simulink model "generic_IVS"  (R2024a)
settings: Solver=FixedStepDiscrete  StartTime=0.0  StopTime=inf  FixedStep=0.001  RelTol=1e-3  EnableMultiTasking=on
model workspace (MAT data in the model file):
  APPROACH = [-49.2532697283 -46.8560638421 -44.4231792578 -41.9812023919 -38.6885385845 -35.362557161 -32.0241539117 -28.6853351363 -25.3485360015 -22.0129625698 -18.6780310991 -15.3435011563 ... (76 elements, 38x2)]
  LANE_LEN = [284; 276; 267]
  LANE_XY = [59.0003214677 62.3317238784 65.6577746803 68.9711287644 72.2614514234 75.5172879138 77.9296982442 80.3117765819 82.6592727002 84.9682672017 87.2351542049 89.4565910317 ... (1704 elements, 284x2x3)]
  N_LANE = 3
  PARK_OCC = [1 1 1 1 1 1 1 1 1 1 1 1 ... (40000 elements, 200x200)]
  WB = 2.9
  branch_lane = 3
  branch_x = -49.2532697283
  branch_y = 17.3349288561
  cruise_lane = 1
  entrance_x = 6
  entrance_y = -36.6
  lane_width = 3.5
  park_goal = [21.4; -44.3; 1.57079632679]
  toll_lane = 1
  toll_post = 20
  toll_pre = 45
  toll_station = 202.6
  toll_x = -176.17
  toll_y = -85.66
  v_cruise = 11
  v_park = 2.78
  waypoints = [-81.8048181182 -79.1416974235 -76.4199514846 -73.3097017696 -70.5703457405 -67.625901331 -64.4903894371 -61.1945301864 -57.8351626085 -54.4642235015 -51.0966947204 -47.7361432477 ... (1754 elements, 877x2)]
libraries: CarMaker4SL x57, simulink x1
(part 2 of 4)

== system generic_IVS/CarMaker ==
  note: Do Not Modify !!
  note: Modify !!
  CM_FIRST : Subsystem
  CM_LAST : Subsystem
  DrivMan : Subsystem
  Ground : Ground
  IPG Vehicle : Subsystem
  IVS_Control : Subsystem
  Subsystem : Subsystem
  Terminator : Terminator
  VehicleControl : Subsystem
  wires:
  DrivMan/2(DrivMan.Out) -> VehicleControl/2(DrivMan.In)
  DrivMan/1(Sync_Out) -> VehicleControl/1(Sync_In)
  CM_FIRST/2(Env.Misc) -> DrivMan/2(Env.Misc)
  CM_FIRST/1(Sync_Out) -> DrivMan/1(Sync_In)
  CM_LAST/1(Sync_Out) -> Terminator/1
  Ground/1 -> CM_FIRST/1(Sync_In)
  IPG Vehicle/1(Sync_Out) -> CM_LAST/1(Sync_In)
  VehicleControl/1(Sync_Out) -> IPG Vehicle/1(Sync_In)
  VehicleControl/3(VhclCtrl.Steering) -> IPG Vehicle/3(VhclCtrl.Steering)
  VehicleControl/4(Vhcl.Wheel.In) -> IPG Vehicle/4(Vhcl.Wheel.In)
  VehicleControl/5(Vhcl.Misc) -> IPG Vehicle/5(Vhcl.Misc)
  VehicleControl/6(VhclCtrl.Brake) -> IPG Vehicle/6(VhclCtrl.Brake)
  VehicleControl/7(VhclCtrl.PT) -> IPG Vehicle/7(VhclCtrl.PT)
  VehicleControl/2(Vhcl.Model.Source) -> IPG Vehicle/2(Vhcl.Model.Source)

== system generic_IVS/Open CarMaker GUI ==
  S-Function : S-Function  FunctionName=cm_gui  SFunctionDeploymentMode=off  EnableBusSupport=off

== system generic_IVS/CarMaker/CM_FIRST ==
  Sync_In : Inport
  BusCreator1 : BusCreator  Inputs=8
  BusCreator2 : BusCreator  Inputs=6
  Demux1 : Demux  Outputs=14
      settings: DisplayOption=none
  Environment : S-Function  FunctionName=CM_Sfun  Parameters='Environment'  SFunctionDeploymentMode=off  EnableBusSupport=off
  IoIn : S-Function  FunctionName=CM_Sfun  Parameters='IoIn'  SFunctionDeploymentMode=off  EnableBusSupport=off
  Terminator : Terminator
  Sync_Out : Outport  VectorParamsAs1DForOutWhenUnconnected=off
  Env.Misc : Outport  Port=2  VectorParamsAs1DForOutWhenUnconnected=off
  wires:
  BusCreator2/1 -> Terminator/1  "IF Environment (in)"
  BusCreator1/1 -> Env.Misc/1
  Demux1/14 -> BusCreator2/6  "Env sRoad"
  Demux1/13 -> BusCreator2/5  "Env PoI_GCS Elev"
  Demux1/12 -> BusCreator2/4  "Env PoI_GCS Lat"
  Demux1/11 -> BusCreator2/3  "Env PoI_GCS Long"
  Demux1/10 -> BusCreator2/2  "Env Time"
  Demux1/9 -> BusCreator2/1  "Env yDay"
  Demux1/8 -> BusCreator1/8  "Env WindVel_tot z"
  Demux1/7 -> BusCreator1/7  "Env WindVel_tot y"
  Demux1/6 -> BusCreator1/6  "Env WindVel_tot x"
  Demux1/5 -> BusCreator1/5  "Env SolarRadiation"
  Demux1/4 -> BusCreator1/4  "Env AirHumidity"
  Demux1/3 -> BusCreator1/3  "Env AirPressure"
  Demux1/2 -> BusCreator1/2  "Env AirDensity"
  Demux1/1 -> BusCreator1/1  "Env Temperature"
  Environment/2 -> Demux1/1
  Environment/1 -> Sync_Out/1
  IoIn/1 -> Environment/1
  Sync_In/1 -> IoIn/1

== system generic_IVS/CarMaker/CM_LAST ==
  Sync_In : Inport
  CM_User : S-Function  FunctionName=CM_Sfun  Parameters='CM_User'  SFunctionDeploymentMode=off  EnableBusSupport=off
  IoOut : S-Function  FunctionName=CM_Sfun  Parameters='IoOut'  SFunctionDeploymentMode=off  EnableBusSupport=off
  Sync_Out : Outport  VectorParamsAs1DForOutWhenUnconnected=off
  wires:
  IoOut/1 -> Sync_Out/1
  CM_User/1 -> IoOut/1
  Sync_In/1 -> CM_User/1

== system generic_IVS/CarMaker/DrivMan ==
  note: There's rarely a reason to override DrivMan signals.
      | Use the VehicleControl interface for this purpose.
  Sync_In : Inport
  Env.Misc : Inport  Port=2
  BusCreator : BusCreator  Inputs=20
  Demux : Demux  Outputs=20
      settings: DisplayOption=none
  DrivMan : S-Function  FunctionName=CM_Sfun  Parameters='DrivMan'  SFunctionDeploymentMode=off  EnableBusSupport=off
  Sync_Out : Outport  VectorParamsAs1DForOutWhenUnconnected=off
  DrivMan.Out : Outport  Port=2  VectorParamsAs1DForOutWhenUnconnected=off
  wires:
  Demux/8 -> BusCreator/8  "DrivMan SelectorCtrl"
  Demux/7 -> BusCreator/7  "DrivMan UserSignal4"
  Demux/6 -> BusCreator/6  "DrivMan UserSignal3"
  Demux/5 -> BusCreator/5  "DrivMan UserSignal2"
  Demux/4 -> BusCreator/4  "DrivMan UserSignal1"
  Demux/3 -> BusCreator/3  "DrivMan UserSignal0"
  Demux/2 -> BusCreator/2  "DrivMan Key"
  Demux/1 -> BusCreator/1  "DrivMan SST"
  Env.Misc/1 -> DrivMan/2
  Sync_In/1 -> DrivMan/1
  DrivMan/1 -> Sync_Out/1
  BusCreator/1 -> DrivMan.Out/1
  DrivMan/2 -> Demux/1
  Demux/9 -> BusCreator/9  "DrivMan DigitalSelectorCtrl0"
  Demux/10 -> BusCreator/10  "DrivMan DigitalSelectorCtrl1"
  Demux/11 -> BusCreator/11  "DrivMan DigitalSelectorCtrl2"
  Demux/20 -> BusCreator/20  "DrivMan Steering Trq"
  Demux/19 -> BusCreator/19  "DrivMan Steering AngAcc"
  Demux/18 -> BusCreator/18  "DrivMan Steering AngVel"
  Demux/17 -> BusCreator/17  "DrivMan Steering Ang"
  Demux/16 -> BusCreator/16  "DrivMan Gas"
  Demux/15 -> BusCreator/15  "DrivMan Clutch"
  Demux/14 -> BusCreator/14  "DrivMan BrakePark"
  Demux/13 -> BusCreator/13  "DrivMan Brake"
  Demux/12 -> BusCreator/12  "DrivMan GearNo"

== system generic_IVS/CarMaker/IPG Vehicle ==
  Sync_In : Inport
  Vhcl.Model.Source : Inport  Port=2
  VhclCtrl.Steering : Inport  Port=3
  Vhcl.Wheel.In : Inport  Port=4
  Vhcl.Misc : Inport  Port=5
  VhclCtrl.Brake : Inport  Port=6
  VhclCtrl.PT : Inport  Port=7
  Brake : Subsystem
  CarAndTrailer : Subsystem
  PowerTrain : Subsystem
  Stop Simulation : Stop
  VehicleSource_BuiltIn : simulink/Logic and Bit Operations/Compare To Constant  relop=~=  const=1  OutDataTypeStr=boolean  ZeroCross=off
  Sync_Out : Outport  VectorParamsAs1DForOutWhenUnconnected=off
  wires:
  VhclCtrl.PT/1 -> PowerTrain/3(VhclCtrl.PT)
  Brake/1(Sync_Out) -> PowerTrain/1(Sync_In)
  CarAndTrailer/1(Sync_Out) -> Brake/1(Sync_In)
  CarAndTrailer/2(Brake.IF.In) -> Brake/2(Brake.IF.In)
  VhclCtrl.Brake/1 -> Brake/3(VhclCtrl.Brake)
  PowerTrain/1(Sync_Out) -> Sync_Out/1
  Vhcl.Misc/1 -> CarAndTrailer/4(Vhcl.Misc)
  Vhcl.Wheel.In/1 -> CarAndTrailer/3(Vhcl.Wheel.In)
  VhclCtrl.Steering/1 -> CarAndTrailer/2(VhclCtrl.Steering)
  Sync_In/1 -> CarAndTrailer/1(Sync_In)
  Vhcl.Model.Source/1 -> VehicleSource_BuiltIn/1
  VehicleSource_BuiltIn/1 -> Stop Simulation/1
  Brake/2(Vhcl.Wheel.PT) -> PowerTrain/2(Vhcl.Wheel.PT)

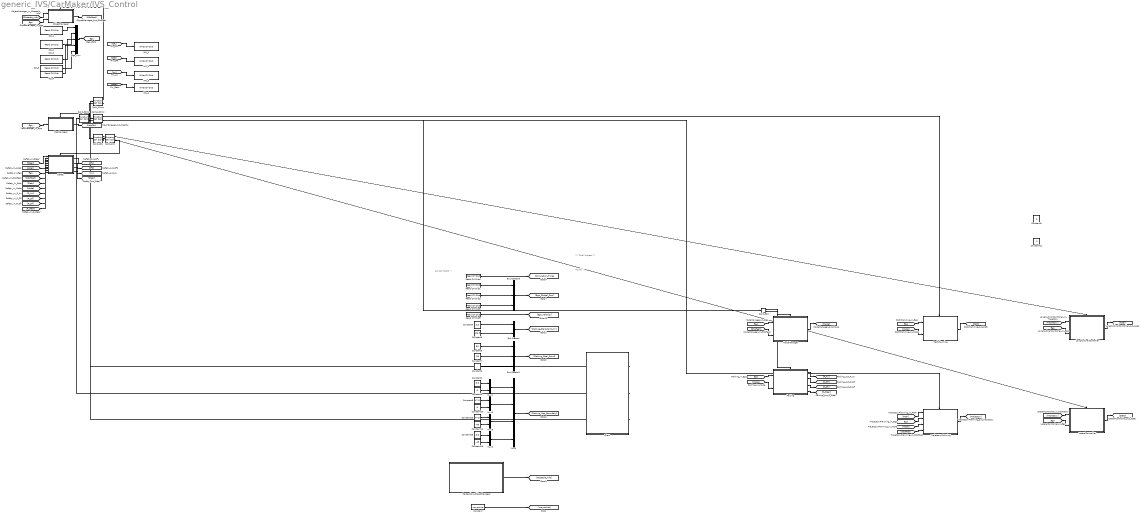
== system generic_IVS/CarMaker/IVS_Control ==
  note: Do Not Modify !!
  note: *** Final Project ***
  note: Modify !!
  Bus Creator : BusCreator  Inputs=2
  Bus Creator1 : BusCreator  Inputs=3
  Bus Creator3 : BusCreator  Inputs=3
  Chart : Stateflow chart  TreatAsAtomicUnit=on
  Constant : Constant  Value=waypoints
  Constant1 : Constant  Value=5.5
  Constant10 : Constant  Value=-4
  Constant11 : Constant  Value=-1
  Constant13 : Constant  Value=47.5
  Constant14 : Constant  Value=-45
  Constant15 : Constant  Value=5.5
  Constant16 : Constant  Value=-45
  Constant2 : Constant  Value=2*pi/3
  Constant3 : Constant
  Constant4 : Constant  Value=5.5
  Constant5 : Constant  Value=-36.5
  Constant6 : Constant  Value=35
  Constant7 : Constant  Value=-30
  Constant8 : Constant  Value=47.5
  Constant9 : Constant  Value=-4
  Ego_Mux : Mux  Inputs=5
  LateralController : Subsystem
  LongitudinalController : Subsystem
  MapManager : Subsystem
  ModeManager : Subsystem
  Mux{2,5,8..9} (4 alike) : Mux  Inputs=2
  Mux4 : Mux
  ObjectManager : Subsystem
  Parking : Subsystem
  PathPlanning : Subsystem
  Perception_ObjectManager : Subsystem
  RD_1 : CarMaker4SL/Read CM Dict  xname=Car.Fr1.tx  xsync=off  xstime=Continuous
  RD_2 : CarMaker4SL/Read CM Dict  xname=Car.Fr1.ty  xsync=off  xstime=Continuous
  RD_3 : CarMaker4SL/Read CM Dict  xname=Car.Fr1.rz  xsync=off  xstime=Continuous
  RD_4 : CarMaker4SL/Read CM Dict  xname=Car.v  xsync=off  xstime=Continuous
  RD_5 : CarMaker4SL/Read CM Dict  xname=Car.Road.sRoad  xsync=off  xstime=Continuous
  Read CM Dict1 : CarMaker4SL/Read CM Dict  xname=Car.Fr1.tx  xsync=off  xstime=Inherited
  Read CM Dict2 : CarMaker4SL/Read CM Dict  xname=Car.Fr1.ty  xsync=off  xstime=Inherited
  Read CM Dict3 : CarMaker4SL/Read CM Dict  xname=Car.Fr1.rz  xsync=off  xstime=Inherited
  Read CM Dict4 : CarMaker4SL/Read CM Dict  xname=Time  xsync=off  xstime=Inherited
  Read CM Dict5 : CarMaker4SL/Read CM Dict  xname=Car.v  xsync=off  xstime=Inherited
  Safety : Subsystem
  Split_100ms : FunctionCallSplit  IconShape=distinctive  NumOutputPorts=2  OutputPortLayout=default
  Split_10b : FunctionCallSplit  IconShape=distinctive  NumOutputPorts=2  OutputPortLayout=default
  Split_10c : FunctionCallSplit  IconShape=distinctive  NumOutputPorts=2  OutputPortLayout=default
  Split_10ms : FunctionCallSplit  IconShape=distinctive  NumOutputPorts=2  OutputPortLayout=default
  Split_50d : FunctionCallSplit  IconShape=distinctive  NumOutputPorts=2  OutputPortLayout=default
  Split_50ms : FunctionCallSplit  IconShape=distinctive  NumOutputPorts=2  OutputPortLayout=default
  TrajectoryPlanning : Subsystem
  WR_1 : CarMaker4SL/Write CM Dict  xname=Car.CFL.rz_ext  xsync=off
  WR_2 : CarMaker4SL/Write CM Dict  xname=Car.CFR.rz_ext  xsync=off
  WR_3 : CarMaker4SL/Write CM Dict  xname=AccelCtrl.DesiredAx  xsync=off
  WR_4 : CarMaker4SL/Write CM Dict  xname=DM.SelectorCtrl  xsync=off
  tag scope: Ego=global
  wires:
  Constant13/1 -> Mux8/1
  Perception_ObjectManager/1(Traffic_Info) -> [Obstacle_Info]
  Read CM Dict1/1 -> Bus Creator3/1  "Car_Fr1_tx"
  Read CM Dict3/1 -> Bus Creator3/3  "Car_Fr1_rz"
  Constant4/1 -> Bus Creator/1  "Parking_Start_Point_X"
  Read CM Dict4/1 -> [Simulation_Time]  "Time"
  Constant9/1 -> Mux2/2
  Bus Creator1/1 -> [Parking_Goal_Point]
  Mux8/1 -> Mux4/3
  Constant6/1 -> Bus Creator1/1  "Parking_Goal_Point_X"
  Constant1/1 -> Mux2/1
  Constant16/1 -> Mux9/2
  Read CM Dict2/1 -> Bus Creator3/2  "Car_Fr1_ty"
  Constant5/1 -> Bus Creator/2  "Parking_Start_Point_Y"
  Constant7/1 -> Bus Creator1/2  "Parking_Goal_Point_Y"
  Read CM Dict5/1 -> [Ego_Velocity]  "Car.v"
  Constant15/1 -> Mux9/1
  Constant10/1 -> Mux5/2
  Bus Creator3/1 -> [Ego_Global_Pos]
  Constant14/1 -> Mux8/2
  Bus Creator/1 -> [Parking_Start_Point_XY]
  Mux9/1 -> Mux4/4
  Mux2/1 -> Mux4/1
  Mux4/1 -> [Parking_Map_Boundary]
  Constant8/1 -> Mux5/1
  Constant2/1 -> Bus Creator1/3  "Parking_Goal_Point_Yaw"
  Mux5/1 -> Mux4/2
  Constant/1 -> [waypoints]
  Chart/1(do_Logic_10ms()) -> Split_10ms/1
  Chart/3(do_Logic_100ms()) -> Split_100ms/1
  RD_1/1 -> Ego_Mux/1
  RD_2/1 -> Ego_Mux/2
  RD_3/1 -> Ego_Mux/3
  RD_4/1 -> Ego_Mux/4
  Ego_Mux/1 -> [Ego]
  Chart/2(do_Logic_50ms()) -> Split_50ms/1
  [Ego] -> MapManager/1(Ego)
  MapManager/1(MapCtx) -> [MapCtx]
  [Trajectory] -> LateralController/1(Trajectory)
  [Ego] -> LateralController/2(Ego)
  LateralController/1(Steer) -> [Steer]
  [Trajectory] -> LongitudinalController/1(Trajectory)
  [Ego] -> LongitudinalController/2(Ego)
  LongitudinalController/1(Accel) -> [Accel]
  Split_50ms/1 -> MapManager/Trigger
  Split_100ms/1 -> PathPlanning/Trigger
  Split_100ms/2 -> TrajectoryPlanning/Trigger
  RD_5/1 -> Ego_Mux/5
  Split_10ms/2 -> Split_10b/1
  [Ego] -> PathPlanning/1(Ego)
  [Mode] -> PathPlanning/2(Mode)
  PathPlanning/1(Path) -> [Path]
  Split_10ms/1 -> ObjectManager/Trigger
  Split_10b/1 -> LateralController/Trigger
  Split_10b/2 -> Split_10c/1
  Split_10c/1 -> LongitudinalController/Trigger
  Split_10c/2 -> Safety/Trigger
  ? -> ?
  ? -> ?
  [Obstacle_Info] -> ObjectManager/1(Obstacle_Info)
  [Ego] -> ObjectManager/2(Ego)
  ObjectManager/1(ObsFeat) -> [ObsFeat]
  [Path] -> TrajectoryPlanning/1(Path)
  [Ego] -> TrajectoryPlanning/2(Ego)
  [Mode] -> TrajectoryPlanning/3(Mode)
  [ObsFeat] -> TrajectoryPlanning/4(ObsFeat)
  TrajectoryPlanning/1(Trajectory) -> [Trajectory]
  [Ego] -> Parking/1(Ego)
  [Mode] -> Parking/2(Mode)
  Parking/1(P_Ax) -> [P_Ax]
  Parking/2(P_Sfl) -> [P_Sfl]
  Parking/3(P_Sfr) -> [P_Sfr]
  Parking/4(P_Gear) -> [P_Gear]
  Split_50ms/2 -> Split_50d/1
  Split_50d/1 -> ModeManager/Trigger
  Split_50d/2 -> Parking/Trigger
  [CFL] -> WR_1/1
  [CFR] -> WR_2/1
  [Ax] -> WR_3/1
  [Gear] -> WR_4/1
  [Steer] -> Safety/1(Steer)
  [Accel] -> Safety/2(Accel)
  [Ego] -> Safety/3(Ego)
  [ObsFeat] -> Safety/4(ObsFeat)
  [Path] -> Safety/5(Path)
  [Mode] -> Safety/6(Mode)
  [P_Ax] -> Safety/7(P_Ax)
  [P_Sfl] -> Safety/8(P_Sfl)
  [P_Sfr] -> Safety/9(P_Sfr)
  [P_Gear] -> Safety/10(P_Gear)
  Safety/1(CFL) -> [CFL]
  Safety/2(CFR) -> [CFR]
  Safety/3(Ax) -> [Ax]
  Safety/4(Gear) -> [Gear]
  [Ego] -> ModeManager/1(Ego)
  [ObsFeat] -> ModeManager/2(ObsFeat)
  ModeManager/1(Mode) -> [Mode]

== system generic_IVS/CarMaker/Subsystem ==
  Day1 : Subsystem  Commented=on
  Day2 : Subsystem  Commented=on
  Day3 : Subsystem  Commented=on
  Day4 & 5 : Subsystem  Commented=on
  Day6 : Subsystem  Commented=on
  Final Project : Subsystem  Commented=on

== system generic_IVS/CarMaker/VehicleControl ==
  note: <Your model here>
  note: When implementing a vehicle control model,
      | be sure to add '-disablevehiclecontrol' to the command line arguments
      | in the CarMaker Model Configuration block.
      | Otherwise your model will possibly not see the original DrivMan signals
      | on its inputs, but those of a currently activated C-coded vehicle control model instead.
  Sync_In : Inport
  DrivMan.In : Inport  Port=2
  Bus Creator2 : BusCreator  Inputs=2
  CreateBus Vhcl.Misc : Subsystem
  CreateBus Vhcl.Wheel.In : Subsystem
  CreateBus VhclCtrl : Subsystem
  CreateBus VhclCtrl.PT : Subsystem
  CreateBus VhclCtrl.Steering : Subsystem
  Demux2 : Demux  Outputs=2
      settings: DisplayOption=none
  VehicleControl : S-Function  FunctionName=CM_Sfun  Parameters='VehicleControl'  SFunctionDeploymentMode=off  EnableBusSupport=off
  VehicleControlUpd : S-Function  FunctionName=CM_Sfun  Parameters='VehicleControlUpd'  SFunctionDeploymentMode=off  EnableBusSupport=off
  Sync_Out : Outport  VectorParamsAs1DForOutWhenUnconnected=off
  Vhcl.Model.Source : Outport  Port=2  VectorParamsAs1DForOutWhenUnconnected=off
  VhclCtrl.Steering : Outport  Port=3  VectorParamsAs1DForOutWhenUnconnected=off
  Vhcl.Wheel.In : Outport  Port=4  VectorParamsAs1DForOutWhenUnconnected=off
  Vhcl.Misc : Outport  Port=5  VectorParamsAs1DForOutWhenUnconnected=off
  VhclCtrl.Brake : Outport  Port=6  VectorParamsAs1DForOutWhenUnconnected=off
  VhclCtrl.PT : Outport  Port=7  VectorParamsAs1DForOutWhenUnconnected=off
  wires:
  CreateBus VhclCtrl/1(Out) -> VehicleControlUpd/2
  VehicleControl/2 -> CreateBus VhclCtrl/1(In)
  VehicleControlUpd/2 -> Vhcl.Model.Source/1
  VehicleControlUpd/4 -> CreateBus Vhcl.Wheel.In/1(In1)
  VehicleControlUpd/5 -> CreateBus Vhcl.Misc/1(In1)
  VehicleControlUpd/6 -> Demux2/1
  VehicleControlUpd/7 -> CreateBus VhclCtrl.PT/1(In1)
  VehicleControlUpd/3 -> CreateBus VhclCtrl.Steering/1(In1)
  CreateBus Vhcl.Misc/1(Out1) -> Vhcl.Misc/1
  CreateBus Vhcl.Wheel.In/1(Out1) -> Vhcl.Wheel.In/1
  DrivMan.In/1 -> VehicleControl/2
  VehicleControl/1 -> VehicleControlUpd/1
  Sync_In/1 -> VehicleControl/1
  CreateBus VhclCtrl.PT/1(Out1) -> VhclCtrl.PT/1
  Bus Creator2/1 -> VhclCtrl.Brake/1
  CreateBus VhclCtrl.Steering/1(Out1) -> VhclCtrl.Steering/1
  VehicleControlUpd/1 -> Sync_Out/1
  Demux2/2 -> Bus Creator2/2  "VhclCtrl BrakePark"
  Demux2/1 -> Bus Creator2/1  "VhclCtrl Brake"

== system generic_IVS/CarMaker/IPG Vehicle/Brake ==
  note: When replacing the entire braking system,
      | be sure to disable the IPG brake model by using the brake
      | model 'Model Manager off' in the vehicle GUI.
  note: <Your model here>
  Sync_In : Inport
  Brake.IF.In : Inport  Port=2
  VhclCtrl.Brake : Inport  Port=3
  Brake : S-Function  FunctionName=CM_Sfun  Parameters='Brake'  SFunctionDeploymentMode=off  EnableBusSupport=off
  BrakeUpd : S-Function  FunctionName=CM_Sfun  Parameters='BrakeUpd'  SFunctionDeploymentMode=off  EnableBusSupport=off
  BusCreator1 : BusCreator  Inputs=16
  CreateBus Vhcl.Wheel.PT : Subsystem
  Demux : Demux  Outputs=16
      settings: DisplayOption=none
  Sync_Out : Outport  VectorParamsAs1DForOutWhenUnconnected=off
  Vhcl.Wheel.PT : Outport  Port=2  VectorParamsAs1DForOutWhenUnconnected=off
  wires:
  Demux/16 -> BusCreator1/16  "Brake IF Trq_DriveSrc_trg d3"
  Demux/15 -> BusCreator1/15  "Brake IF Trq_DriveSrc_trg d2"
  Demux/14 -> BusCreator1/14  "Brake IF Trq_DriveSrc_trg d1"
  Demux/13 -> BusCreator1/13  "Brake IF Trq_DriveSrc_trg d0"
  Demux/12 -> BusCreator1/12  "Brake IF Trq_Reg_trg RR"
  Demux/11 -> BusCreator1/11  "Brake IF Trq_Reg_trg RL"
  Demux/10 -> BusCreator1/10  "Brake IF Trq_Reg_trg FR"
  Demux/9 -> BusCreator1/9  "Brake IF Trq_Reg_trg FL"
  Demux/8 -> BusCreator1/8  "Brake IF Trq_PB RR"
  Demux/7 -> BusCreator1/7  "Brake IF Trq_PB RL"
  Demux/6 -> BusCreator1/6  "Brake IF Trq_PB FR"
  Demux/5 -> BusCreator1/5  "Brake IF Trq_PB FL"
  Demux/4 -> BusCreator1/4  "Brake IF Trq_WB RR"
  Demux/3 -> BusCreator1/3  "Brake IF Trq_WB RL"
  Demux/2 -> BusCreator1/2  "Brake IF Trq_WB FR"
  Demux/1 -> BusCreator1/1  "Brake IF Trq_WB FL"
  Brake/2 -> Demux/1
  BusCreator1/1 -> BrakeUpd/2
  BrakeUpd/1 -> Sync_Out/1
  Brake/1 -> BrakeUpd/1  "Sync"
  Brake.IF.In/1 -> Brake/2
  VhclCtrl.Brake/1 -> Brake/3
  Sync_In/1 -> Brake/1
  BrakeUpd/2 -> CreateBus Vhcl.Wheel.PT/1(In)
  CreateBus Vhcl.Wheel.PT/1(Out) -> Vhcl.Wheel.PT/1

== system generic_IVS/CarMaker/IPG Vehicle/CarAndTrailer ==
  Sync_In : Inport
  VhclCtrl.Steering : Inport  Port=2
  Vhcl.Wheel.In : Inport  Port=3
  Vhcl.Misc : Inport  Port=4
  CarAndTrailerUpd : Subsystem
  Forces : Subsystem
  Ground : Ground
  Kinematics : Subsystem
  Kinetics : Subsystem
  Steering : Subsystem
  Terminator : Terminator
  Terminator1 : Terminator
  Trailer : Subsystem
  Sync_Out : Outport  VectorParamsAs1DForOutWhenUnconnected=off
  Brake.IF.In : Outport  Port=2  VectorParamsAs1DForOutWhenUnconnected=off
  wires:
  Trailer/9(Car.Hitch.FrcTrq) -> CarAndTrailerUpd/9(Car.Hitch.FrcTrq)
  Trailer/8(Vhcl.Wheel.RR) -> CarAndTrailerUpd/8(Vhcl.Wheel.RR)
  Trailer/7(Vhcl.Wheel.RL) -> CarAndTrailerUpd/7(Vhcl.Wheel.RL)
  Trailer/6(Vhcl.Wheel.FR) -> CarAndTrailerUpd/6(Vhcl.Wheel.FR)
  Trailer/5(Vhcl.Wheel.FL) -> CarAndTrailerUpd/5(Vhcl.Wheel.FL)
  Trailer/4(Vhcl.PoI) -> CarAndTrailerUpd/4(Vhcl.PoI)
  Trailer/3(Vhcl.Motion) -> CarAndTrailerUpd/3(Vhcl.Motion)
  Trailer/2(Vhcl.Steering) -> CarAndTrailerUpd/2(Vhcl.Steering)
  Trailer/1(Sync_Out) -> CarAndTrailerUpd/1(Sync_In)
  CarAndTrailerUpd/2(Brake.IF.In) -> Brake.IF.In/1
  CarAndTrailerUpd/1(Sync_Out) -> Sync_Out/1
  Vhcl.Misc/1 -> Terminator1/1
  Vhcl.Wheel.In/1 -> Terminator/1
  Kinetics/6(WheelCarrier.Misc) -> Trailer/6(WheelCarrier.Misc)
  Kinetics/5(Car.Trq_T2W) -> Trailer/5(Car.Trq_T2W)
  Steering/2(Steer.IF) -> Kinematics/2(Steer.IF)
  Kinetics/4(Car.Fr1) -> Trailer/4(Car.Fr1)
  Kinetics/3(Car.Hitch) -> Trailer/3(Car.Hitch)
  Kinetics/2(Trailer.Load) -> Trailer/2(Trailer.Load)
  VhclCtrl.Steering/1 -> Steering/2(VhclCtrl.Steering)
  Sync_In/1 -> Steering/1(Sync_In)
  Steering/1(Sync_Out) -> Kinematics/1(Sync_In)
  Kinetics/1(Sync_Out) -> Trailer/1(Sync_In)
  Ground/1 -> CarAndTrailerUpd/10(Vhcl.Fr1A)
  Forces/8(TireRR_Out) -> Kinetics/8(TireRR.Out)
  Forces/7(TireRL_Out) -> Kinetics/7(TireRL.Out)
  Forces/6(TireFR_Out) -> Kinetics/6(TireFR.Out)
  Forces/5(TireFL_Out) -> Kinetics/5(TireFL.Out)
  Forces/4(Car.Load) -> Kinetics/4(Car.Load)
  Forces/2(Car.Virtual) -> Kinetics/2(Car.Virtual)
  Kinematics/6(lSpring) -> Forces/6(lSpring)
  Kinematics/7(vDamp) -> Forces/7(vDamp)
  Forces/3(Car.Aero) -> Kinetics/3(Car.Aero)
  Forces/1(Sync_Out) -> Kinetics/1(Sync_In)
  Kinematics/5(TireRR_In) -> Forces/5(TireRR_In)
  Kinematics/4(TireRL_In) -> Forces/4(TireRL_In)
  Kinematics/3(TireFR_In) -> Forces/3(TireFR_In)
  Kinematics/2(TireFL_In) -> Forces/2(TireFL_In)
  Kinematics/1(Sync_Out) -> Forces/1(Sync_In)
  Kinematics/8(lStabi) -> Forces/8(lStabi)
  Kinematics/9(lBuf) -> Forces/9(lBuf)

== system generic_IVS/CarMaker/IPG Vehicle/PowerTrain ==
  note: When replacing the entire powertrain,
      | be sure to disable the IPG powertrain model by using the powertrain
      | model 'Model Manager off' in the vehicle GUI.
  note: <Your model here>
  Sync_In : Inport
  Vhcl.Wheel.PT : Inport  Port=2
  VhclCtrl.PT : Inport  Port=3
  BusCreator1 : BusCreator  Inputs=42
  Demux1 : Demux  Outputs=42
      settings: DisplayOption=none
  PowerTrain : S-Function  FunctionName=CM_Sfun  Parameters='PowerTrain'  SFunctionDeploymentMode=off  EnableBusSupport=off
  PowerTrainUpd : S-Function  FunctionName=CM_Sfun  Parameters='PowerTrainUpd'  SFunctionDeploymentMode=off  EnableBusSupport=off
  Sync_Out : Outport  VectorParamsAs1DForOutWhenUnconnected=off
  wires:
  BusCreator1/1 -> PowerTrainUpd/2
  Demux1/42 -> BusCreator1/42  "PT IF WRR Trq_BrakeReg_max"
  Demux1/41 -> BusCreator1/41  "PT IF WRR Trq_BrakeReg"
  Demux1/40 -> BusCreator1/40  "PT IF WRR Trq_Supp2WC"
  Demux1/39 -> BusCreator1/39  "PT IF WRR Trq_Drive"
  Demux1/38 -> BusCreator1/38  "PT IF WRR Trq_B2W"
  Demux1/37 -> BusCreator1/37  "PT IF WRR rotv"
  Demux1/36 -> BusCreator1/36  "PT IF WRR rot"
  Demux1/35 -> BusCreator1/35  "PT IF WRL Trq_BrakeReg_max"
  Demux1/34 -> BusCreator1/34  "PT IF WRL Trq_BrakeReg"
  Demux1/33 -> BusCreator1/33  "PT IF WRL Trq_Supp2WC"
  Demux1/32 -> BusCreator1/32  "PT IF WRL Trq_Drive"
  Demux1/31 -> BusCreator1/31  "PT IF WRL Trq_B2W"
  Demux1/30 -> BusCreator1/30  "PT IF WRL rotv"
  Demux1/29 -> BusCreator1/29  "PT IF WRL rot"
  Demux1/28 -> BusCreator1/28  "PT IF WFR Trq_BrakeReg_max"
  Demux1/27 -> BusCreator1/27  "PT IF WFR Trq_BrakeReg"
  Demux1/26 -> BusCreator1/26  "PT IF WFR Trq_Supp2WC"
  Demux1/25 -> BusCreator1/25  "PT IF WFR Trq_Drive"
  Demux1/24 -> BusCreator1/24  "PT IF WFR Trq_B2W"
  Demux1/23 -> BusCreator1/23  "PT IF WFR rotv"
  Demux1/22 -> BusCreator1/22  "PT IF WFR rot"
  Demux1/21 -> BusCreator1/21  "PT IF WFL Trq_BrakeReg_max"
  Demux1/20 -> BusCreator1/20  "PT IF WFL Trq_BrakeReg"
  Demux1/19 -> BusCreator1/19  "PT IF WFL Trq_Supp2WC"
  Demux1/18 -> BusCreator1/18  "PT IF WFL Trq_Drive"
  Demux1/17 -> BusCreator1/17  "PT IF WFL Trq_B2W"
  Demux1/16 -> BusCreator1/16  "PT IF WFL rotv"
  Demux1/15 -> BusCreator1/15  "PT IF WFL rot"
  Demux1/14 -> BusCreator1/14  "PT IF DL_iDiff_mean"
  Demux1/13 -> BusCreator1/13  "PT IF Trq_Supp2BdyEng y"
  Demux1/12 -> BusCreator1/12  "PT IF Trq_Supp2BdyEng x"
  Demux1/11 -> BusCreator1/11  "PT IF Trq_Supp2Bdy1B z"
  Demux1/10 -> BusCreator1/10  "PT IF Trq_Supp2Bdy1B y"
  Demux1/9 -> BusCreator1/9  "PT IF Trq_Supp2Bdy1B x"
  Demux1/8 -> BusCreator1/8  "PT IF Trq_Supp2Bdy1 z"
  Demux1/7 -> BusCreator1/7  "PT IF Trq_Supp2Bdy1 y"
  Demux1/6 -> BusCreator1/6  "PT IF Trq_Supp2Bdy1 x"
  Demux1/5 -> BusCreator1/5  "PT IF Engine_rotv"
  Demux1/4 -> BusCreator1/4  "PT IF GearNo"
  Demux1/3 -> BusCreator1/3  "PT IF OperationError"
  Demux1/2 -> BusCreator1/2  "PT IF OperationState"
  Demux1/1 -> BusCreator1/1  "PT IF Ignition"
  Sync_In/1 -> PowerTrain/1
  PowerTrain/2 -> Demux1/1
  PowerTrainUpd/1 -> Sync_Out/1
  PowerTrain/1 -> PowerTrainUpd/1  "Sync"
  VhclCtrl.PT/1 -> PowerTrain/3
  Vhcl.Wheel.PT/1 -> PowerTrain/2

== system generic_IVS/CarMaker/IVS_Control/LateralController ==
  Trajectory : Inport
  Ego : Inport  Port=2
  Trigger : TriggerPort  TriggerType=function-call  VariantControl=(inherit)
  P_3 : Constant  Value=WB
  latctrl : MATLAB Function  TreatAsAtomicUnit=on
  Steer : Outport
  wires:
  Trajectory/1 -> latctrl/1(Traj)
  Ego/1 -> latctrl/2(Ego)
  P_3/1 -> latctrl/3(WB)
  latctrl/1(steer) -> Steer/1

== system generic_IVS/CarMaker/IVS_Control/LongitudinalController ==
  Trajectory : Inport
  Ego : Inport  Port=2
  Trigger : TriggerPort  TriggerType=function-call  VariantControl=(inherit)
  lonctrl : MATLAB Function  TreatAsAtomicUnit=on
  Accel : Outport
  wires:
  Trajectory/1 -> lonctrl/1(Traj)
  Ego/1 -> lonctrl/2(Ego)
  lonctrl/1(ax) -> Accel/1

== system generic_IVS/CarMaker/IVS_Control/MapManager ==
  Ego : Inport
  Trigger : TriggerPort  TriggerType=function-call  VariantControl=(inherit)
  P_2 : Constant  Value=LANE_XY
  P_3 : Constant  Value=LANE_LEN
  mapmgr : MATLAB Function  TreatAsAtomicUnit=on
  MapCtx : Outport
  wires:
  Ego/1 -> mapmgr/1(Ego)
  P_2/1 -> mapmgr/2(LANE_XY)
  P_3/1 -> mapmgr/3(LANE_LEN)
  mapmgr/1(MapCtx) -> MapCtx/1

== system generic_IVS/CarMaker/IVS_Control/ModeManager ==
  Ego : Inport
  ObsFeat : Inport  Port=2
  Trigger : TriggerPort  TriggerType=function-call  VariantControl=(inherit)
  P_10 : Constant  Value=toll_lane
  P_11 : Constant  Value=toll_x
  P_12 : Constant  Value=toll_y
  P_13 : Constant  Value=branch_x
  P_14 : Constant  Value=branch_y
  P_15 : Constant  Value=entrance_x
  P_16 : Constant  Value=entrance_y
  P_3 : Constant  Value=LANE_XY
  P_4 : Constant  Value=LANE_LEN
  P_5 : Constant  Value=cruise_lane
  P_6 : Constant  Value=v_cruise
  P_7 : Constant  Value=v_park
  P_8 : Constant  Value=lane_width
  P_9 : Constant  Value=branch_lane
  modemgr : MATLAB Function  TreatAsAtomicUnit=on
  Mode : Outport
  wires:
  Ego/1 -> modemgr/1(Ego)
  ObsFeat/1 -> modemgr/2(OF)
  P_3/1 -> modemgr/3(LANE_XY)
  P_4/1 -> modemgr/4(LANE_LEN)
  P_5/1 -> modemgr/5(cruise_lane)
  P_6/1 -> modemgr/6(v_cruise)
  P_7/1 -> modemgr/7(v_park)
  P_8/1 -> modemgr/8(lane_width)
  P_9/1 -> modemgr/9(branch_lane)
  P_10/1 -> modemgr/10(toll_lane)
  P_11/1 -> modemgr/11(toll_x)
  P_12/1 -> modemgr/12(toll_y)
  P_13/1 -> modemgr/13(branch_x)
  P_14/1 -> modemgr/14(branch_y)
  P_15/1 -> modemgr/15(entrance_x)
  P_16/1 -> modemgr/16(entrance_y)
  modemgr/1(Mode) -> Mode/1

== system generic_IVS/CarMaker/IVS_Control/ObjectManager ==
  Obstacle_Info : Inport
  Ego : Inport  Port=2
  Trigger : TriggerPort  TriggerType=function-call  VariantControl=(inherit)
  objmgr : MATLAB Function  TreatAsAtomicUnit=on
  ObsFeat : Outport
  wires:
  Obstacle_Info/1 -> objmgr/1(Obs)
  Ego/1 -> objmgr/2(Ego)
  objmgr/1(ObsFeat) -> ObsFeat/1

== system generic_IVS/CarMaker/IVS_Control/Parking ==
  Ego : Inport
  Mode : Inport  Port=2
  Trigger : TriggerPort  TriggerType=function-call  VariantControl=(inherit)
  P_3 : Constant  Value=park_goal
  P_4 : Constant  Value=PARK_OCC
  parking_wrap : MATLAB Function  TreatAsAtomicUnit=on
  P_Ax : Outport
  P_Sfl : Outport  Port=2
  P_Sfr : Outport  Port=3
  P_Gear : Outport  Port=4
  wires:
  Ego/1 -> parking_wrap/1(Ego)
  Mode/1 -> parking_wrap/2(Mode)
  P_3/1 -> parking_wrap/3(goal)
  P_4/1 -> parking_wrap/4(occ)
  parking_wrap/1(ax) -> P_Ax/1
  parking_wrap/2(sfl) -> P_Sfl/1
  parking_wrap/3(sfr) -> P_Sfr/1
  parking_wrap/4(gear) -> P_Gear/1

== system generic_IVS/CarMaker/IVS_Control/PathPlanning ==
  Ego : Inport
  Mode : Inport  Port=2
  Trigger : TriggerPort  TriggerType=function-call  VariantControl=(inherit)
  P_3 : Constant  Value=LANE_XY
  P_4 : Constant  Value=LANE_LEN
  P_5 : Constant  Value=[-49.25327 17.33493;-46.85606 15.84163;-44.42318 15.19366;-41.9812 14.60087;-38.68854 14.01143;-35.36256 13.6848;-32.02415 13.5706;-28.68534 13.58386;-25.34854 13.64604;-22.01296 13.70953;-18.67803 13.75912;-15.3435 13.79135;-12.00923 13.80761;-8.675115 13.81141;-6.844851 12.65834;-4.475925 11.2828;-2.929245 9.699698;-1.787116 7.705912;-1.091386 5.377188;-0.8039891 2.068424;-0.9063824 -0.8655854;-1.112701 -3.98989;-1.277334 -7.230635;-1.362389 -10.52727;-1.393461 -13.81922;-1.387211 -17.05992;-1.381831 -20.19758;-1.387521 -23.69495;-1.356218 -26.77355;-1.171809 -29.643;-0.6361997 -32.35289;0.4595539 -34.84087;1.819229 -36.64147;2.8 -36.6;3.8 -36.6;4.8 -36.6;5.8 -36.6;6.8 -36.6]
  pathplan : MATLAB Function  TreatAsAtomicUnit=on
  Path : Outport
  wires:
  Ego/1 -> pathplan/1(Ego)
  Mode/1 -> pathplan/2(Mode)
  P_3/1 -> pathplan/3(LANE_XY)
  P_4/1 -> pathplan/4(LANE_LEN)
  P_5/1 -> pathplan/5(APPROACH)
  pathplan/1(Path) -> Path/1

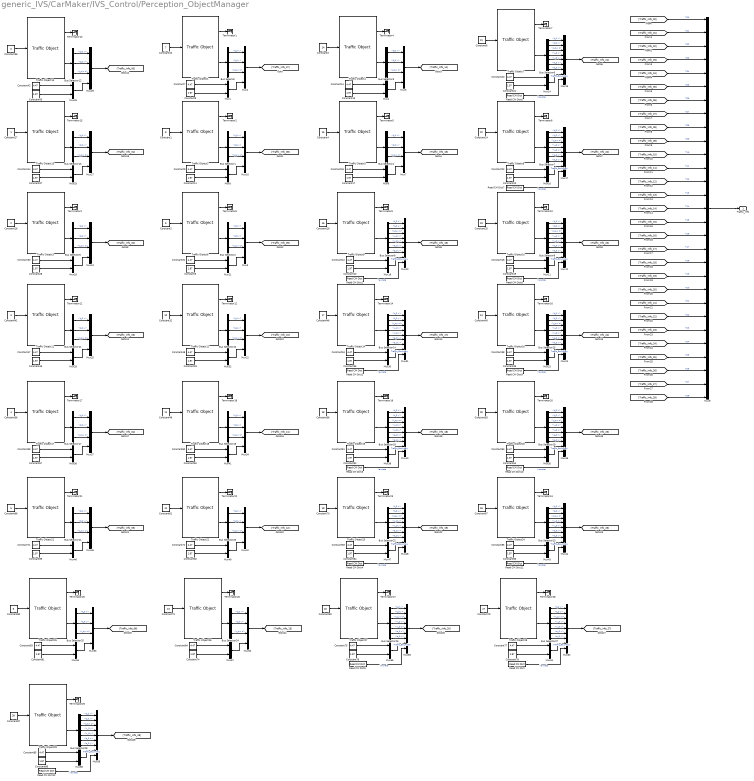
== system generic_IVS/CarMaker/IVS_Control/Perception_ObjectManager ==
  Bus Selector{,1..5,10..13,16..17,20..21,24..25} (16 alike) : BusSelector  OutputSignals=t_0 x,t_0 y,r_zyx z
  Bus Selector{6..9,14..15,18..19,22..23,26..28} (13 alike) : BusSelector  OutputSignals=t_0 x,t_0 y,r_zyx z,v_0 x,v_0 y,a_0 x,a_0 y
  Constant1 : Constant  Value=8
  Constant10 : Constant  Value=7
  Constant{5,8,11,13,15,17,19,21,23,28,33,35,37,39,43,45,50,52,54,57,62,64,66,69,74,76,78,81,86} (29 alike) : Constant  Value=1.97
  Constant{7,9,12,14,16,18,20,22,30..31,34,38,42,44,47..48,51,53,59..60,63,65,71..72,75,77,83..85} (29 alike) : Constant  Value=4.47
  Constant2 : Constant  Value=9
  Constant24 : Constant  Value=22
  Constant25 : Constant  Value=23
  Constant26 : Constant  Value=2
  Constant27 : Constant
  Constant29 : Constant  Value=16
  Constant3 : Constant  Value=14
  Constant32 : Constant  Value=10
  Constant36 : Constant  Value=0
  Constant4 : Constant  Value=15
  Constant40 : Constant  Value=24
  Constant41 : Constant  Value=3
  Constant46 : Constant  Value=17
  Constant49 : Constant  Value=11
  Constant55 : Constant  Value=25
  Constant56 : Constant  Value=4
  Constant58 : Constant  Value=18
  Constant6 : Constant  Value=21
  Constant61 : Constant  Value=12
  Constant67 : Constant  Value=26
  Constant68 : Constant  Value=5
  Constant70 : Constant  Value=19
  Constant73 : Constant  Value=13
  Constant79 : Constant  Value=27
  Constant80 : Constant  Value=6
  Constant82 : Constant  Value=20
  Constant87 : Constant  Value=28
  Mux{1,4,6,8,11,14,16,18..19,21,23,26,28,30,32..33,35,38..39,41,43,46..47,49,51,54..55,57..58} (29 alike) : Mux  Inputs=2
  Mux{2..3,5,7,10,13,22,25,27,29,34,37,42,45,50,53} (16 alike) : Mux
  Mux{12,15,17,20,24,31,36,40,44,48,52,56,59} (13 alike) : Mux  Inputs=9
  Mux9 : Mux  Inputs=29
  Read CM Dict : CarMaker4SL/Read CM Dict  xname=Traffic.T27.rzv  xsync=off  xstime=Continuous
  Read CM Dict1 : CarMaker4SL/Read CM Dict  xname=Traffic.T16.rzv  xsync=off  xstime=Continuous
  Read CM Dict10 : CarMaker4SL/Read CM Dict  xname=Traffic.T25.rzv  xsync=off  xstime=Continuous
  Read CM Dict11 : CarMaker4SL/Read CM Dict  xname=Traffic.T26.rzv  xsync=off  xstime=Continuous
  Read CM Dict12 : CarMaker4SL/Read CM Dict  xname=Traffic.T28.rzv  xsync=off  xstime=Continuous
  Read CM Dict2 : CarMaker4SL/Read CM Dict  xname=Traffic.T17.rzv  xsync=off  xstime=Continuous
  Read CM Dict3 : CarMaker4SL/Read CM Dict  xname=Traffic.T18.rzv  xsync=off  xstime=Continuous
  Read CM Dict4 : CarMaker4SL/Read CM Dict  xname=Traffic.T19.rzv  xsync=off  xstime=Continuous
  Read CM Dict5 : CarMaker4SL/Read CM Dict  xname=Traffic.T20.rzv  xsync=off  xstime=Continuous
  Read CM Dict6 : CarMaker4SL/Read CM Dict  xname=Traffic.T21.rzv  xsync=off  xstime=Continuous
  Read CM Dict7 : CarMaker4SL/Read CM Dict  xname=Traffic.T22.rzv  xsync=off  xstime=Continuous
  Read CM Dict8 : CarMaker4SL/Read CM Dict  xname=Traffic.T23.rzv  xsync=off  xstime=Continuous
  Read CM Dict9 : CarMaker4SL/Read CM Dict  xname=Traffic.T24.rzv  xsync=off  xstime=Continuous
  Terminator{1..29} (29 alike) : Terminator
  Traffic Object1 : CarMaker4SL/Traffic Object  xname=T07  ximode=Traffic Id  xstime=Inherited
      settings: SourceProductName=CarMaker4SL
  Traffic Object10 : CarMaker4SL/Traffic Object  xname=T23  ximode=Traffic Id  xstime=Inherited
      settings: SourceProductName=CarMaker4SL
  Traffic Object11 : CarMaker4SL/Traffic Object  xname=T03  ximode=Traffic Id  xstime=Inherited
      settings: SourceProductName=CarMaker4SL
  Traffic Object12 : CarMaker4SL/Traffic Object  xname=T10  ximode=Traffic Id  xstime=Inherited
      settings: SourceProductName=CarMaker4SL
  Traffic Object13 : CarMaker4SL/Traffic Object  xname=T00  ximode=Traffic Id  xstime=Inherited
      settings: SourceProductName=CarMaker4SL
  Traffic Object14 : CarMaker4SL/Traffic Object  xname=T17  ximode=Traffic Id  xstime=Inherited
      settings: SourceProductName=CarMaker4SL
  Traffic Object15 : CarMaker4SL/Traffic Object  xname=T01  ximode=Traffic Id  xstime=Inherited
      settings: SourceProductName=CarMaker4SL
  Traffic Object16 : CarMaker4SL/Traffic Object  xname=T24  ximode=Traffic Id  xstime=Inherited
      settings: SourceProductName=CarMaker4SL
  Traffic Object17 : CarMaker4SL/Traffic Object  xname=T04  ximode=Traffic Id  xstime=Inherited
      settings: SourceProductName=CarMaker4SL
  Traffic Object18 : CarMaker4SL/Traffic Object  xname=T11  ximode=Traffic Id  xstime=Inherited
      settings: SourceProductName=CarMaker4SL
  Traffic Object19 : CarMaker4SL/Traffic Object  xname=T18  ximode=Traffic Id  xstime=Inherited
      settings: SourceProductName=CarMaker4SL
  Traffic Object2 : CarMaker4SL/Traffic Object  xname=T08  ximode=Traffic Id  xstime=Inherited
      settings: SourceProductName=CarMaker4SL
  Traffic Object20 : CarMaker4SL/Traffic Object  xname=T25  ximode=Traffic Id  xstime=Inherited
      settings: SourceProductName=CarMaker4SL
  Traffic Object21 : CarMaker4SL/Traffic Object  xname=T05  ximode=Traffic Id  xstime=Inherited
      settings: SourceProductName=CarMaker4SL
  Traffic Object22 : CarMaker4SL/Traffic Object  xname=T12  ximode=Traffic Id  xstime=Inherited
      settings: SourceProductName=CarMaker4SL
  Traffic Object23 : CarMaker4SL/Traffic Object  xname=T19  ximode=Traffic Id  xstime=Inherited
      settings: SourceProductName=CarMaker4SL
  Traffic Object24 : CarMaker4SL/Traffic Object  xname=T26  ximode=Traffic Id  xstime=Inherited
      settings: SourceProductName=CarMaker4SL
  Traffic Object25 : CarMaker4SL/Traffic Object  xname=T06  ximode=Traffic Id  xstime=Inherited
      settings: SourceProductName=CarMaker4SL
  Traffic Object26 : CarMaker4SL/Traffic Object  xname=T13  ximode=Traffic Id  xstime=Inherited
      settings: SourceProductName=CarMaker4SL
  Traffic Object27 : CarMaker4SL/Traffic Object  xname=T20  ximode=Traffic Id  xstime=Inherited
      settings: SourceProductName=CarMaker4SL
  Traffic Object28 : CarMaker4SL/Traffic Object  xname=T27  ximode=Traffic Id  xstime=Inherited
      settings: SourceProductName=CarMaker4SL
  Traffic Object29 : CarMaker4SL/Traffic Object  xname=T28  ximode=Traffic Id  xstime=Inherited
      settings: SourceProductName=CarMaker4SL
  Traffic Object3 : CarMaker4SL/Traffic Object  xname=T02  ximode=Traffic Id  xstime=Inherited
      settings: SourceProductName=CarMaker4SL
  Traffic Object4 : CarMaker4SL/Traffic Object  xname=T14  ximode=Traffic Id  xstime=Inherited
      settings: SourceProductName=CarMaker4SL
  Traffic Object5 : CarMaker4SL/Traffic Object  xname=T15  ximode=Traffic Id  xstime=Inherited
      settings: SourceProductName=CarMaker4SL
  Traffic Object6 : CarMaker4SL/Traffic Object  xname=T09  ximode=Traffic Id  xstime=Inherited
      settings: SourceProductName=CarMaker4SL
  Traffic Object7 : CarMaker4SL/Traffic Object  xname=T21  ximode=Traffic Id  xstime=Inherited
      settings: SourceProductName=CarMaker4SL
  Traffic Object8 : CarMaker4SL/Traffic Object  xname=T22  ximode=Traffic Id  xstime=Inherited
      settings: SourceProductName=CarMaker4SL
  Traffic Object9 : CarMaker4SL/Traffic Object  xname=T16  ximode=Traffic Id  xstime=Inherited
      settings: SourceProductName=CarMaker4SL
  Traffic_Info : Outport
  wires:
  Mux9/1 -> Traffic_Info/1
  Traffic Object29/1 -> Terminator29/1
  Bus Selector28/1 -> Mux59/1  "<t_0 x>"
  Bus Selector28/2 -> Mux59/2  "<t_0 y>"
  Bus Selector28/4 -> Mux59/4  "<v_0 x>"
  Constant87/1 -> Traffic Object29/1
  Traffic Object29/2 -> Bus Selector28/1
  Constant86/1 -> Mux58/2
  Mux59/1 -> [Traffic_Info_28]
  Constant85/1 -> Mux58/1
  Bus Selector28/3 -> Mux59/3  "<r_zyx z>"
  Bus Selector28/6 -> Mux59/6  "<a_0 x>"
  Bus Selector28/7 -> Mux59/7  "<a_0 y>"
  Bus Selector28/5 -> Mux59/5  "<v_0 y>"
  Read CM Dict12/1 -> Mux59/9  "Yawrate"
  Mux58/1 -> Mux59/8  "Traffic_Boundary"
  Traffic Object24/1 -> Terminator24/1
  Bus Selector23/1 -> Mux44/1  "<t_0 x>"
  Bus Selector23/2 -> Mux44/2  "<t_0 y>"
  Bus Selector23/4 -> Mux44/4  "<v_0 x>"
  Constant67/1 -> Traffic Object24/1
  Traffic Object24/2 -> Bus Selector23/1
  Constant66/1 -> Mux43/2
  Mux44/1 -> [Traffic_Info_26]
  Constant65/1 -> Mux43/1
  Bus Selector23/3 -> Mux44/3  "<r_zyx z>"
  Bus Selector23/6 -> Mux44/6  "<a_0 x>"
  Bus Selector23/7 -> Mux44/7  "<a_0 y>"
  Bus Selector23/5 -> Mux44/5  "<v_0 y>"
  Read CM Dict11/1 -> Mux44/9  "Yawrate"
  Mux43/1 -> Mux44/8  "Traffic_Boundary"
  Traffic Object20/1 -> Terminator20/1
  Bus Selector19/1 -> Mux36/1  "<t_0 x>"
  Bus Selector19/2 -> Mux36/2  "<t_0 y>"
  Bus Selector19/4 -> Mux36/4  "<v_0 x>"
  Constant55/1 -> Traffic Object20/1
  Traffic Object20/2 -> Bus Selector19/1
  Constant54/1 -> Mux35/2
  Mux36/1 -> [Traffic_Info_25]
  Constant53/1 -> Mux35/1
  Bus Selector19/3 -> Mux36/3  "<r_zyx z>"
  Bus Selector19/6 -> Mux36/6  "<a_0 x>"
  Bus Selector19/7 -> Mux36/7  "<a_0 y>"
  Bus Selector19/5 -> Mux36/5  "<v_0 y>"
  Read CM Dict10/1 -> Mux36/9  "Yawrate"
  Mux35/1 -> Mux36/8  "Traffic_Boundary"
  Traffic Object16/1 -> Terminator16/1
  Bus Selector15/1 -> Mux24/1  "<t_0 x>"
  Bus Selector15/2 -> Mux24/2  "<t_0 y>"
  Bus Selector15/4 -> Mux24/4  "<v_0 x>"
  Constant40/1 -> Traffic Object16/1
  Traffic Object16/2 -> Bus Selector15/1
  Constant39/1 -> Mux23/2
  Mux24/1 -> [Traffic_Info_24]
  Constant38/1 -> Mux23/1
  Bus Selector15/3 -> Mux24/3  "<r_zyx z>"
  Bus Selector15/6 -> Mux24/6  "<a_0 x>"
  Bus Selector15/7 -> Mux24/7  "<a_0 y>"
  Bus Selector15/5 -> Mux24/5  "<v_0 y>"
  Read CM Dict9/1 -> Mux24/9  "Yawrate"
  Mux23/1 -> Mux24/8  "Traffic_Boundary"
  Traffic Object10/1 -> Terminator10/1
  Bus Selector9/1 -> Mux12/1  "<t_0 x>"
  Bus Selector9/2 -> Mux12/2  "<t_0 y>"
  Bus Selector9/4 -> Mux12/4  "<v_0 x>"
  Constant25/1 -> Traffic Object10/1
  Traffic Object10/2 -> Bus Selector9/1
  Constant19/1 -> Mux11/2
  Mux12/1 -> [Traffic_Info_23]
  Constant18/1 -> Mux11/1
  Bus Selector9/3 -> Mux12/3  "<r_zyx z>"
  Bus Selector9/6 -> Mux12/6  "<a_0 x>"
  Bus Selector9/7 -> Mux12/7  "<a_0 y>"
  Bus Selector9/5 -> Mux12/5  "<v_0 y>"
  Read CM Dict8/1 -> Mux12/9  "Yawrate"
  Mux11/1 -> Mux12/8  "Traffic_Boundary"
  Traffic Object8/1 -> Terminator8/1
  Bus Selector7/1 -> Mux17/1  "<t_0 x>"
  Bus Selector7/2 -> Mux17/2  "<t_0 y>"
  Bus Selector7/4 -> Mux17/4  "<v_0 x>"
  Constant24/1 -> Traffic Object8/1
  Traffic Object8/2 -> Bus Selector7/1
  Constant23/1 -> Mux16/2
  Mux17/1 -> [Traffic_Info_22]
  Constant22/1 -> Mux16/1
  Bus Selector7/3 -> Mux17/3  "<r_zyx z>"
  Bus Selector7/6 -> Mux17/6  "<a_0 x>"
  Bus Selector7/7 -> Mux17/7  "<a_0 y>"
  Bus Selector7/5 -> Mux17/5  "<v_0 y>"
  Read CM Dict7/1 -> Mux17/9  "Yawrate"
  Mux16/1 -> Mux17/8  "Traffic_Boundary"
  Traffic Object7/1 -> Terminator7/1
  Bus Selector6/1 -> Mux15/1  "<t_0 x>"
  Bus Selector6/2 -> Mux15/2  "<t_0 y>"
  Bus Selector6/4 -> Mux15/4  "<v_0 x>"
  Constant6/1 -> Traffic Object7/1
  Traffic Object7/2 -> Bus Selector6/1
  Constant21/1 -> Mux14/2
  Mux15/1 -> [Traffic_Info_21]
  Constant20/1 -> Mux14/1
  Bus Selector6/3 -> Mux15/3  "<r_zyx z>"
  Bus Selector6/6 -> Mux15/6  "<a_0 x>"
  Bus Selector6/7 -> Mux15/7  "<a_0 y>"
  Bus Selector6/5 -> Mux15/5  "<v_0 y>"
  Read CM Dict6/1 -> Mux15/9  "Yawrate"
  Mux14/1 -> Mux15/8  "Traffic_Boundary"
  Traffic Object27/1 -> Terminator27/1
  Bus Selector26/1 -> Mux56/1  "<t_0 x>"
  Bus Selector26/2 -> Mux56/2  "<t_0 y>"
  Bus Selector26/4 -> Mux56/4  "<v_0 x>"
  Constant82/1 -> Traffic Object27/1
  Traffic Object27/2 -> Bus Selector26/1
  Constant76/1 -> Mux55/2
  Mux56/1 -> [Traffic_Info_20]
  Constant75/1 -> Mux55/1
  Bus Selector26/3 -> Mux56/3  "<r_zyx z>"
  Bus Selector26/6 -> Mux56/6  "<a_0 x>"
  Bus Selector26/7 -> Mux56/7  "<a_0 y>"
  Bus Selector26/5 -> Mux56/5  "<v_0 y>"
  Read CM Dict5/1 -> Mux56/9  "Yawrate"
  Mux55/1 -> Mux56/8  "Traffic_Boundary"
  Traffic Object23/1 -> Terminator23/1
  Bus Selector22/1 -> Mux48/1  "<t_0 x>"
  Bus Selector22/2 -> Mux48/2  "<t_0 y>"
  Bus Selector22/4 -> Mux48/4  "<v_0 x>"
  Constant70/1 -> Traffic Object23/1
  Traffic Object23/2 -> Bus Selector22/1
  Constant64/1 -> Mux47/2
  Mux48/1 -> [Traffic_Info_19]
  Constant63/1 -> Mux47/1
  Bus Selector22/3 -> Mux48/3  "<r_zyx z>"
  Bus Selector22/6 -> Mux48/6  "<a_0 x>"
  Bus Selector22/7 -> Mux48/7  "<a_0 y>"
  Bus Selector22/5 -> Mux48/5  "<v_0 y>"
  Read CM Dict4/1 -> Mux48/9  "Yawrate"
  Mux47/1 -> Mux48/8  "Traffic_Boundary"
  Traffic Object19/1 -> Terminator19/1
  Bus Selector18/1 -> Mux40/1  "<t_0 x>"
  Bus Selector18/2 -> Mux40/2  "<t_0 y>"
  Bus Selector18/4 -> Mux40/4  "<v_0 x>"
  Constant58/1 -> Traffic Object19/1
  Traffic Object19/2 -> Bus Selector18/1
  Constant52/1 -> Mux39/2
  Mux40/1 -> [Traffic_Info_18]
  Constant51/1 -> Mux39/1
  Bus Selector18/3 -> Mux40/3  "<r_zyx z>"
  Bus Selector18/6 -> Mux40/6  "<a_0 x>"
  Bus Selector18/7 -> Mux40/7  "<a_0 y>"
  Bus Selector18/5 -> Mux40/5  "<v_0 y>"
  Read CM Dict3/1 -> Mux40/9  "Yawrate"
  Mux39/1 -> Mux40/8  "Traffic_Boundary"
  Traffic Object14/1 -> Terminator14/1
  Bus Selector14/1 -> Mux31/1  "<t_0 x>"
  Bus Selector14/2 -> Mux31/2  "<t_0 y>"
  Bus Selector14/4 -> Mux31/4  "<v_0 x>"
  Constant46/1 -> Traffic Object14/1
  Traffic Object14/2 -> Bus Selector14/1
  Constant35/1 -> Mux30/2
  Mux31/1 -> [Traffic_Info_17]
  Constant34/1 -> Mux30/1
  Bus Selector14/3 -> Mux31/3  "<r_zyx z>"
  Bus Selector14/6 -> Mux31/6  "<a_0 x>"
  Bus Selector14/7 -> Mux31/7  "<a_0 y>"
  Bus Selector14/5 -> Mux31/5  "<v_0 y>"
  Read CM Dict2/1 -> Mux31/9  "Yawrate"
  Mux30/1 -> Mux31/8  "Traffic_Boundary"
  Traffic Object9/1 -> Terminator9/1
  Bus Selector8/1 -> Mux20/1  "<t_0 x>"
  Bus Selector8/2 -> Mux20/2  "<t_0 y>"
  Bus Selector8/4 -> Mux20/4  "<v_0 x>"
  Constant29/1 -> Traffic Object9/1
  Traffic Object9/2 -> Bus Selector8/1
  Constant13/1 -> Mux19/2
  Mux20/1 -> [Traffic_Info_16]
  Constant12/1 -> Mux19/1
  Bus Selector8/3 -> Mux20/3  "<r_zyx z>"
  Bus Selector8/6 -> Mux20/6  "<a_0 x>"
  Bus Selector8/7 -> Mux20/7  "<a_0 y>"
  Bus Selector8/5 -> Mux20/5  "<v_0 y>"
  Read CM Dict1/1 -> Mux20/9  "Yawrate"
  Mux19/1 -> Mux20/8  "Traffic_Boundary"
  Read CM Dict/1 -> Mux52/9  "Yawrate"
  Mux51/1 -> Mux52/8  "Traffic_Boundary"
  Bus Selector27/7 -> Mux52/7  "<a_0 y>"
  Bus Selector27/6 -> Mux52/6  "<a_0 x>"
  Bus Selector27/5 -> Mux52/5  "<v_0 y>"
  Bus Selector27/4 -> Mux52/4  "<v_0 x>"
  [Traffic_Info_28] -> Mux9/29  "T28"
  Constant10/1 -> Traffic Object1/1
  Traffic Object1/1 -> Terminator1/1
  Traffic Object2/1 -> Terminator2/1
  Constant1/1 -> Traffic Object2/1
  Traffic Object4/1 -> Terminator4/1
  Constant3/1 -> Traffic Object4/1
  Constant4/1 -> Traffic Object5/1
  Traffic Object5/1 -> Terminator5/1
  Traffic Object1/2 -> Bus Selector/1
  Bus Selector/1 -> Mux2/1  "<t_0 x>"
  Bus Selector/2 -> Mux2/2  "<t_0 y>"
  Bus Selector/3 -> Mux2/3  "<r_zyx z>"
  Bus Selector1/2 -> Mux10/2  "<t_0 y>"
  Mux10/1 -> [Traffic_Info_08]
  Bus Selector1/1 -> Mux10/1  "<t_0 x>"
  Bus Selector1/3 -> Mux10/3  "<r_zyx z>"
  Traffic Object2/2 -> Bus Selector1/1
  Bus Selector3/2 -> Mux5/2  "<t_0 y>"
  Mux5/1 -> [Traffic_Info_14]
  Bus Selector3/1 -> Mux5/1  "<t_0 x>"
  Bus Selector3/3 -> Mux5/3  "<r_zyx z>"
  Traffic Object4/2 -> Bus Selector3/1
  Bus Selector4/2 -> Mux7/2  "<t_0 y>"
  Mux7/1 -> [Traffic_Info_15]
  Bus Selector4/1 -> Mux7/1  "<t_0 x>"
  Bus Selector4/3 -> Mux7/3  "<r_zyx z>"
  Traffic Object5/2 -> Bus Selector4/1
  Mux2/1 -> [Traffic_Info_07]
  [Traffic_Info_00] -> Mux9/1  "T00"
  [Traffic_Info_01] -> Mux9/2  "T01"
  [Traffic_Info_02] -> Mux9/3  "T02"
  [Traffic_Info_06] -> Mux9/7  "T06"
  [Traffic_Info_05] -> Mux9/6  "T05"
  [Traffic_Info_04] -> Mux9/5  "T04"
  [Traffic_Info_03] -> Mux9/4  "T03"
  Constant8/1 -> Mux1/2
  Mux1/1 -> Mux2/4
  Constant7/1 -> Mux1/1
  Constant11/1 -> Mux8/2
  Constant9/1 -> Mux8/1
  Mux8/1 -> Mux10/4
  Constant15/1 -> Mux4/2
  Constant14/1 -> Mux4/1
  Mux4/1 -> Mux5/4
  Constant17/1 -> Mux6/2
  Constant16/1 -> Mux6/1
  Mux6/1 -> Mux7/4
  Constant37/1 -> Mux33/2
  Traffic Object13/2 -> Bus Selector12/1
  Mux26/1 -> Mux29/4
  Bus Selector12/1 -> Mux29/1  "<t_0 x>"
  Constant36/1 -> Traffic Object13/1
  Constant42/1 -> Mux26/1
  Mux27/1 -> [Traffic_Info_01]
  Traffic Object15/2 -> Bus Selector13/1
  Traffic Object13/1 -> Terminator13/1
  Traffic Object15/1 -> Terminator15/1
  Bus Selector12/2 -> Mux29/2  "<t_0 y>"
  Constant44/1 -> Mux33/1
  Bus Selector13/1 -> Mux27/1  "<t_0 x>"
  Mux33/1 -> Mux27/4
  Bus Selector13/3 -> Mux27/3  "<r_zyx z>"
  Bus Selector13/2 -> Mux27/2  "<t_0 y>"
  Constant43/1 -> Mux26/2
  Mux29/1 -> [Traffic_Info_00]
  Bus Selector12/3 -> Mux29/3  "<r_zyx z>"
  Constant27/1 -> Traffic Object15/1
  Constant5/1 -> Mux21/2
  Constant26/1 -> Traffic Object3/1
  Bus Selector5/2 -> Mux13/2  "<t_0 y>"
  Mux3/1 -> [Traffic_Info_09]
  Bus Selector2/2 -> Mux3/2  "<t_0 y>"
  Mux21/1 -> Mux3/4
  Traffic Object6/2 -> Bus Selector2/1
  Bus Selector2/1 -> Mux3/1  "<t_0 x>"
  Traffic Object6/1 -> Terminator6/1
  Bus Selector2/3 -> Mux3/3  "<r_zyx z>"
  Constant28/1 -> Mux18/2
  Traffic Object3/2 -> Bus Selector5/1
  Traffic Object3/1 -> Terminator3/1
  Mux13/1 -> [Traffic_Info_02]
  Bus Selector5/3 -> Mux13/3  "<r_zyx z>"
  Constant2/1 -> Traffic Object6/1
  Bus Selector5/1 -> Mux13/1  "<t_0 x>"
  Mux18/1 -> Mux13/4
  Constant30/1 -> Mux18/1
  Constant31/1 -> Mux21/1
  Constant33/1 -> Mux32/2
  Constant41/1 -> Traffic Object11/1
  Bus Selector11/2 -> Mux25/2  "<t_0 y>"
  Mux22/1 -> [Traffic_Info_10]
  Bus Selector10/2 -> Mux22/2  "<t_0 y>"
  Mux32/1 -> Mux22/4
  Traffic Object12/2 -> Bus Selector10/1
  Bus Selector10/1 -> Mux22/1  "<t_0 x>"
  Traffic Object12/1 -> Terminator12/1
  Bus Selector10/3 -> Mux22/3  "<r_zyx z>"
  Constant45/1 -> Mux28/2
  Traffic Object11/2 -> Bus Selector11/1
  Traffic Object11/1 -> Terminator11/1
  Mux25/1 -> [Traffic_Info_03]
  Bus Selector11/3 -> Mux25/3  "<r_zyx z>"
  Constant32/1 -> Traffic Object12/1
  Bus Selector11/1 -> Mux25/1  "<t_0 x>"
  Mux28/1 -> Mux25/4
  Constant47/1 -> Mux28/1
  Constant48/1 -> Mux32/1
  Constant50/1 -> Mux41/2
  Constant56/1 -> Traffic Object17/1
  Bus Selector17/2 -> Mux37/2  "<t_0 y>"
  Mux34/1 -> [Traffic_Info_11]
  Bus Selector16/2 -> Mux34/2  "<t_0 y>"
  Mux41/1 -> Mux34/4
  Traffic Object18/2 -> Bus Selector16/1
  Bus Selector16/1 -> Mux34/1  "<t_0 x>"
  Traffic Object18/1 -> Terminator18/1
  Bus Selector16/3 -> Mux34/3  "<r_zyx z>"
  Constant57/1 -> Mux38/2
  Traffic Object17/2 -> Bus Selector17/1
  Traffic Object17/1 -> Terminator17/1
  Mux37/1 -> [Traffic_Info_04]
  Bus Selector17/3 -> Mux37/3  "<r_zyx z>"
  Constant49/1 -> Traffic Object18/1
  Bus Selector17/1 -> Mux37/1  "<t_0 x>"
  Mux38/1 -> Mux37/4
  Constant59/1 -> Mux38/1
  Constant60/1 -> Mux41/1
  Constant62/1 -> Mux49/2
  Constant68/1 -> Traffic Object21/1
  Bus Selector21/2 -> Mux45/2  "<t_0 y>"
  Mux42/1 -> [Traffic_Info_12]
  Bus Selector20/2 -> Mux42/2  "<t_0 y>"
  Mux49/1 -> Mux42/4
  Traffic Object22/2 -> Bus Selector20/1
  Bus Selector20/1 -> Mux42/1  "<t_0 x>"
  Traffic Object22/1 -> Terminator22/1
  Bus Selector20/3 -> Mux42/3  "<r_zyx z>"
  Constant69/1 -> Mux46/2
  Traffic Object21/2 -> Bus Selector21/1
  Traffic Object21/1 -> Terminator21/1
  Mux45/1 -> [Traffic_Info_05]
  Bus Selector21/3 -> Mux45/3  "<r_zyx z>"
  Constant61/1 -> Traffic Object22/1
  Bus Selector21/1 -> Mux45/1  "<t_0 x>"
  Mux46/1 -> Mux45/4
  Constant71/1 -> Mux46/1
  Constant72/1 -> Mux49/1
  Constant79/1 -> Traffic Object28/1
  Mux52/1 -> [Traffic_Info_27]
  Bus Selector27/1 -> Mux52/1  "<t_0 x>"
  Constant78/1 -> Mux51/2
  Traffic Object28/2 -> Bus Selector27/1
  Constant77/1 -> Mux51/1
  Bus Selector27/3 -> Mux52/3  "<r_zyx z>"
  Constant74/1 -> Mux57/2
  Constant80/1 -> Traffic Object25/1
  Bus Selector25/2 -> Mux53/2  "<t_0 y>"
  Mux50/1 -> [Traffic_Info_13]
  Bus Selector27/2 -> Mux52/2  "<t_0 y>"
  Bus Selector24/2 -> Mux50/2  "<t_0 y>"
  Mux57/1 -> Mux50/4
  Traffic Object26/2 -> Bus Selector24/1
  Bus Selector24/1 -> Mux50/1  "<t_0 x>"
  Traffic Object26/1 -> Terminator26/1
  Bus Selector24/3 -> Mux50/3  "<r_zyx z>"
  Constant81/1 -> Mux54/2
  Traffic Object25/2 -> Bus Selector25/1
  Traffic Object25/1 -> Terminator25/1
  Traffic Object28/1 -> Terminator28/1
  Mux53/1 -> [Traffic_Info_06]
  Bus Selector25/3 -> Mux53/3  "<r_zyx z>"
  Constant73/1 -> Traffic Object26/1
  Bus Selector25/1 -> Mux53/1  "<t_0 x>"
  Mux54/1 -> Mux53/4
  Constant83/1 -> Mux54/1
  Constant84/1 -> Mux57/1
  [Traffic_Info_09] -> Mux9/10  "T09"
  [Traffic_Info_10] -> Mux9/11  "T10"
  [Traffic_Info_11] -> Mux9/12  "T11"
  [Traffic_Info_08] -> Mux9/9  "T08"
  [Traffic_Info_12] -> Mux9/13  "T12"
  [Traffic_Info_13] -> Mux9/14  "T13"
  [Traffic_Info_07] -> Mux9/8  "T07"
  [Traffic_Info_16] -> Mux9/17  "T16"
  [Traffic_Info_17] -> Mux9/18  "T17"
  [Traffic_Info_18] -> Mux9/19  "T18"
  [Traffic_Info_15] -> Mux9/16  "T15"
  [Traffic_Info_19] -> Mux9/20  "T19"
  [Traffic_Info_20] -> Mux9/21  "T20"
  [Traffic_Info_14] -> Mux9/15  "T14"
  [Traffic_Info_23] -> Mux9/24  "T23"
  [Traffic_Info_24] -> Mux9/25  "T24"
  [Traffic_Info_25] -> Mux9/26  "T25"
  [Traffic_Info_22] -> Mux9/23  "T22"
  [Traffic_Info_26] -> Mux9/27  "T26"
  [Traffic_Info_27] -> Mux9/28  "T27"
  [Traffic_Info_21] -> Mux9/22  "T21"
